simulink model "sampleModel1896"  (R2023a)
settings: Solver=VariableStepAuto  StartTime=0.0  StopTime=10.0  RelTol=1e-3
libraries: hdlsllib x5
settings Model: Creator=user1  LastModifiedBy=user1

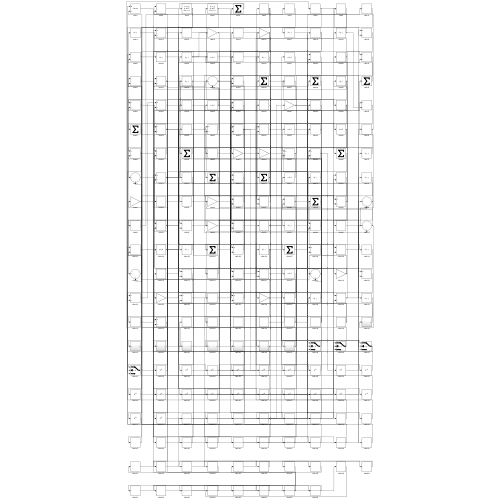
[thumbnail: Simulink's stored preview of the top-level diagram]
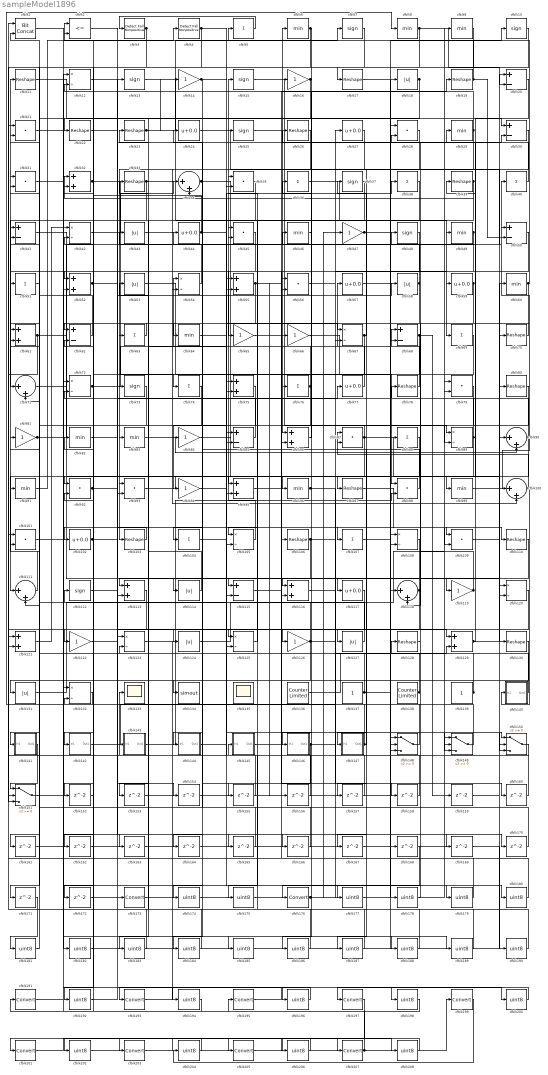
== system sampleModel1896 ==
  cfblk1 : hdlsllib/Logic and Bit Operations/Bit Concat  numInputs=2
  cfblk{7,10,13,15,25,37,48,73,112} (9 alike) : Signum
  cfblk{34,71,90,100,111,118} (6 alike) : Sum  Inputs=|++
  cfblk{21,28,31,35,45,56,79,87,92..93,98,101,109} (13 alike) : DotProduct  OutDataTypeStr=Inherit: Inherit via internal rule
  cfblk{24,27,44,57,59,77,102,117} (8 alike) : Bias  Bias=0.0  SaturateOnIntegerOverflow=off
  cfblk{11,17,19,22..23,26,33,39,70,78,80,97,103,106,110,128,130} (17 alike) : Reshape
  cfblk{5,36,38,40,51,63,69,74,76,88,104,107} (12 alike) : Sum  Inputs=+
  cfblk{12,42,54,67,72,89,105,108,120,123,125,132} (12 alike) : Product  Inputs=*/  RndMeth=Zero  SaturateOnIntegerOverflow=on
  cfblk{32,52,55,61,75,86,95,113,116,121,129} (11 alike) : Sum
  cfblk{18,43,53,58,114,124,127,131} (8 alike) : Abs  SaturateOnIntegerOverflow=off
  cfblk{20,30,41,50,62,68,85,115} (8 alike) : Sum  Inputs=+-
  cfblk{14,16,47,65..66,81,84,94,119,122,126} (11 alike) : Gain
  cfblk133 : Scope
  cfblk134 : ToWorkspace  VariableName=simout  SaveFormat=Timeseries  SampleTime=-1
  cfblk135 : Scope
      settings: Floating=on
  cfblk136 : hdlsllib/Sources/Counter Limited  uplimit=7  tsamp=-1
  cfblk137 : Constant  SampleTime=-1
  cfblk138 : hdlsllib/Sources/Counter Limited  uplimit=7  tsamp=-1
  cfblk139 : Constant  SampleTime=-1
  cfblk140 : Subsystem
      settings: LibrarySourceBlock=|
      | hdlsllib/Ports &
      | Subsystems/Subsystem
  cfblk141 : Subsystem
      settings: LibrarySourceBlock=|
      | hdlsllib/Ports &
      | Subsystems/Subsystem
  cfblk142 : Subsystem
      settings: LibrarySourceBlock=|
      | hdlsllib/Ports &
      | Subsystems/Subsystem
  cfblk143 : Subsystem
      settings: LibrarySourceBlock=|
      | hdlsllib/Ports &
      | Subsystems/Subsystem
  cfblk144 : Subsystem
      settings: LibrarySourceBlock=|
      | hdlsllib/Ports &
      | Subsystems/Subsystem
  cfblk145 : Subsystem
      settings: LibrarySourceBlock=|
      | hdlsllib/Ports &
      | Subsystems/Subsystem
  cfblk146 : Subsystem
      settings: LibrarySourceBlock=|
      | hdlsllib/Ports &
      | Subsystems/Subsystem
  cfblk147 : Subsystem
      settings: LibrarySourceBlock=|
      | hdlsllib/Ports &
      | Subsystems/Subsystem
  cfblk{148..151} (4 alike) : Switch  SaturateOnIntegerOverflow=off  InputSameDT=off
  cfblk{152..172} (21 alike) : Delay  SampleTime=1
  cfblk{173,176,191,193,195,197,199,201,203,205,207} (11 alike) : DataTypeConversion  SaturateOnIntegerOverflow=off  RndMeth=Floor
  cfblk{174..175,177..190,192,194,196,198,200,202,204,206,208} (25 alike) : DataTypeConversion  OutDataTypeStr=uint8  SaturateOnIntegerOverflow=off  RndMeth=Floor
  cfblk2 : RelationalOperator  Operator=<=  OutDataTypeStr=boolean  InputSameDT=off
  cfblk{6,8..9,29,46,49,60,64,82..83,91,96,99} (13 alike) : MinMax
  cfblk3 : hdlsllib/Logic and Bit Operations/Detect Fall Nonpositive  vinit=0  OutDataTypeStr=boolean
  cfblk4 : hdlsllib/Logic and Bit Operations/Detect Fall Nonpositive  vinit=0  OutDataTypeStr=boolean
  wires:
  cfblk68/1 -> cfblk105/2, cfblk159/1
  cfblk54/1 -> cfblk22/1
  cfblk32/1 -> cfblk74/1, cfblk162/1
  cfblk105/1 -> cfblk15/1
  cfblk98/1 -> cfblk44/1
  cfblk121/1 -> cfblk42/1
  cfblk128/1 -> cfblk57/1
  cfblk30/1 -> cfblk108/2
  cfblk91/1 -> cfblk4/1
  cfblk84/1 -> cfblk96/1
  cfblk53/1 -> cfblk98/1
  cfblk137/1 -> cfblk18/1, cfblk32/1
  cfblk26/1 -> cfblk103/1
  cfblk114/1 -> cfblk53/1
  cfblk61/1 -> cfblk115/1, cfblk121/2
  cfblk70/1 -> cfblk63/1
  cfblk93/1 -> cfblk95/1
  cfblk34/1 -> cfblk148/2, cfblk120/2
  cfblk25/1 -> cfblk86/1
  cfblk5/1 -> cfblk3/1
  cfblk138/1 -> cfblk48/1, cfblk134/1, cfblk81/1
  cfblk60/1 -> cfblk5/1, cfblk118/2
  cfblk99/1 -> cfblk40/1
  cfblk23/1 -> cfblk7/1, cfblk14/1, cfblk30/2
  cfblk41/1 -> cfblk97/1
  cfblk92/1 -> cfblk13/1, cfblk107/1
  cfblk81/1 -> cfblk20/1, cfblk61/2
  cfblk111/1 -> cfblk11/1
  cfblk20/1 -> cfblk99/1
  cfblk49/1 -> cfblk65/1, cfblk45/2
  cfblk71/1 -> cfblk119/1
  cfblk97/1 -> cfblk110/1
  cfblk9/1 -> cfblk126/1
  cfblk89/1 -> cfblk39/1, cfblk144/1(In1), cfblk36/1
  cfblk87/1 -> cfblk130/1, cfblk104/1, cfblk84/1
  cfblk17/1 -> cfblk89/1
  cfblk140/1(Out1) -> cfblk78/1
  cfblk15/1 -> cfblk89/2
  cfblk8/1 -> cfblk20/2, cfblk113/2
  cfblk145/1(Out1) -> cfblk106/1
  cfblk28/1 -> cfblk176/1
  cfblk55/1 -> cfblk73/1, cfblk19/1, cfblk114/1, cfblk156/1
  cfblk64/1 -> cfblk95/2
  cfblk96/1 -> cfblk50/1, cfblk150/2
  cfblk36/1 -> cfblk69/1
  cfblk90/1 -> cfblk43/1, cfblk157/1
  cfblk109/1 -> cfblk80/1
  cfblk150/1 -> cfblk133/1
  cfblk100/1 -> cfblk140/1(In1), cfblk87/2
  cfblk73/1 -> cfblk83/1
  cfblk76/1 -> cfblk23/1, cfblk116/2
  cfblk63/1 -> cfblk62/1
  cfblk13/1 -> cfblk88/1
  cfblk77/1 -> cfblk54/1
  cfblk40/1 -> cfblk6/1
  cfblk125/1 -> cfblk45/1
  cfblk35/1 -> cfblk71/1
  cfblk119/1 -> cfblk116/1, cfblk68/2
  cfblk118/1 -> cfblk117/1, cfblk151/3
  cfblk115/1 -> cfblk98/2
  cfblk124/1 -> cfblk9/1
  cfblk50/1 -> cfblk86/2
  cfblk122/1 -> cfblk46/1
  cfblk127/1 -> cfblk112/1
  cfblk38/1 -> cfblk125/1
  cfblk129/1 -> cfblk60/1, cfblk29/1
  cfblk106/1 -> cfblk113/1, cfblk149/3, cfblk153/1
  cfblk45/1 -> cfblk51/1
  cfblk131/1 -> cfblk75/1
  cfblk112/1 -> cfblk77/1
  cfblk48/1 -> cfblk125/2
  cfblk42/1 -> cfblk34/1
  cfblk88/1 -> cfblk111/1
  cfblk10/1 -> cfblk17/1
  cfblk142/1(Out1) -> cfblk27/1
  cfblk46/1 -> cfblk146/1(In1)
  cfblk108/1 -> cfblk127/1
  cfblk148/1 -> cfblk33/1
  cfblk58/1 -> cfblk92/1, cfblk24/1
  cfblk75/1 -> cfblk94/1
  cfblk146/1(Out1) -> cfblk129/2, cfblk164/1
  cfblk132/1 -> cfblk8/1
  cfblk102/1 -> cfblk129/1, cfblk124/1, cfblk170/1
  cfblk4/1 -> cfblk141/1(In1), cfblk67/1
  cfblk86/1 -> cfblk16/1
  cfblk33/1 -> cfblk85/2, cfblk172/1
  cfblk83/1 -> cfblk90/2
  cfblk51/1 -> cfblk91/1
  cfblk72/1 -> cfblk55/2, cfblk58/1, cfblk25/1
  cfblk47/1 -> cfblk49/1, cfblk169/1
  cfblk67/1 -> cfblk122/1, cfblk37/1
  cfblk29/1 -> cfblk12/2, cfblk167/1
  cfblk78/1 -> cfblk35/1
  cfblk44/1 -> cfblk2/1, cfblk150/3
  cfblk82/1 -> cfblk109/1
  cfblk59/1 -> cfblk105/1, cfblk187/1
  cfblk19/1 -> cfblk2/2, cfblk50/2
  cfblk27/1 -> cfblk54/2
  cfblk147/1(Out1) -> cfblk31/1, cfblk87/1
  cfblk104/1 -> cfblk75/2
  cfblk37/1 -> cfblk93/1
  cfblk65/1 -> cfblk26/1
  cfblk18/1 -> cfblk41/1, cfblk52/2
  cfblk7/1 -> cfblk142/1(In1)
  cfblk136/1 -> cfblk128/1
  cfblk130/1 -> cfblk131/1
  cfblk39/1 -> cfblk93/2, cfblk32/2
  cfblk62/1 -> cfblk41/2
  cfblk141/1(Out1) -> cfblk151/1
  cfblk85/1 -> cfblk72/2
  cfblk56/1 -> cfblk59/1
  cfblk24/1 -> cfblk120/1
  cfblk144/1(Out1) -> cfblk38/1
  cfblk126/1 -> cfblk71/2, cfblk150/1, cfblk171/1
  cfblk3/1 -> cfblk52/1, cfblk151/2
  cfblk52/1 -> cfblk143/1(In1), cfblk166/1
  cfblk143/1(Out1) -> cfblk66/1
  cfblk6/1 -> cfblk111/2, cfblk61/1, cfblk76/1
  cfblk103/1 -> cfblk102/1
  cfblk16/1 -> cfblk35/2, cfblk184/1
  cfblk110/1 -> cfblk147/1(In1)
  cfblk149/1 -> cfblk132/2
  cfblk139/1 -> cfblk68/1, cfblk92/2
  cfblk11/1 -> cfblk30/1
  cfblk107/1 -> cfblk10/1
  cfblk2/1 -> cfblk109/2
  cfblk66/1 -> cfblk118/1
  cfblk14/1 -> cfblk115/2, cfblk64/1
  cfblk43/1 -> cfblk100/2
  cfblk113/1 -> cfblk152/1
  cfblk152/1 -> cfblk62/2
  cfblk153/1 -> cfblk56/2
  cfblk22/1 -> cfblk154/1
  cfblk154/1 -> cfblk108/1
  cfblk80/1 -> cfblk155/1
  cfblk155/1 -> cfblk132/1
  cfblk156/1 -> cfblk85/1
  cfblk157/1 -> cfblk55/1
  cfblk116/1 -> cfblk158/1
  cfblk158/1 -> cfblk121/1
  cfblk159/1 -> cfblk90/1
  cfblk95/1 -> cfblk160/1
  cfblk160/1 -> cfblk72/1
  cfblk74/1 -> cfblk161/1
  cfblk161/1 -> cfblk148/1
  cfblk162/1 -> cfblk149/2
  cfblk151/1 -> cfblk163/1
  cfblk163/1 -> cfblk149/1
  cfblk164/1 -> cfblk100/1
  cfblk12/1 -> cfblk165/1
  cfblk165/1 -> cfblk42/2
  cfblk166/1 -> cfblk34/2
  cfblk170/1 -> cfblk31/2
  cfblk172/1 -> cfblk148/3
  cfblk117/1 -> cfblk174/1
  cfblk174/1 -> cfblk79/1
  cfblk120/1 -> cfblk175/1
  cfblk175/1 -> cfblk79/2
  cfblk176/1 -> cfblk67/2, cfblk47/1
  cfblk94/1 -> cfblk177/1
  cfblk177/1 -> cfblk28/1
  cfblk57/1 -> cfblk178/1
  cfblk178/1 -> cfblk28/2
  cfblk1/1 -> cfblk179/1
  cfblk179/1 -> cfblk56/1
  cfblk167/1 -> cfblk180/1
  cfblk180/1 -> cfblk1/1
  cfblk171/1 -> cfblk181/1
  cfblk181/1 -> cfblk1/2
  cfblk101/1 -> cfblk182/1
  cfblk182/1 -> cfblk168/1
  cfblk69/1 -> cfblk183/1
  cfblk183/1 -> cfblk101/1
  cfblk184/1 -> cfblk101/2
  cfblk21/1 -> cfblk185/1
  cfblk185/1 -> cfblk70/1
  cfblk168/1 -> cfblk186/1
  cfblk186/1 -> cfblk21/1
  cfblk187/1 -> cfblk21/2
  cfblk123/1 -> cfblk188/1
  cfblk188/1 -> cfblk145/1(In1)
  cfblk31/1 -> cfblk189/1
  cfblk189/1 -> cfblk123/1
  cfblk169/1 -> cfblk190/1
  cfblk190/1 -> cfblk123/2
  cfblk79/1 -> cfblk192/1
  cfblk192/1 -> cfblk173/1
  cfblk173/1 -> cfblk194/1
  cfblk194/1 -> cfblk191/1
  cfblk191/1 -> cfblk196/1
  cfblk196/1 -> cfblk193/1
  cfblk193/1 -> cfblk198/1
  cfblk198/1 -> cfblk195/1
  cfblk195/1 -> cfblk200/1
  cfblk200/1 -> cfblk197/1
  cfblk197/1 -> cfblk202/1
  cfblk202/1 -> cfblk199/1
  cfblk199/1 -> cfblk204/1
  cfblk204/1 -> cfblk201/1
  cfblk205/1 -> cfblk207/1
  cfblk201/1 -> cfblk206/1
  cfblk206/1 -> cfblk203/1
  cfblk207/1 -> cfblk82/1, cfblk12/1
  cfblk203/1 -> cfblk208/1
  cfblk208/1 -> cfblk205/1

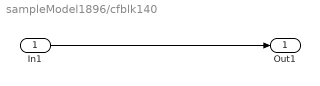
== system sampleModel1896/cfblk140 ==
  In1 : Inport
  Out1 : Outport
  wires:
  In1/1 -> Out1/1

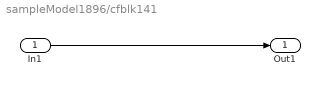
== system sampleModel1896/cfblk141 ==
  In1 : Inport
  Out1 : Outport
  wires:
  In1/1 -> Out1/1

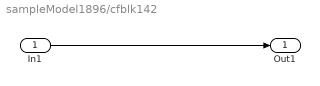
== system sampleModel1896/cfblk142 ==
  In1 : Inport
  Out1 : Outport
  wires:
  In1/1 -> Out1/1

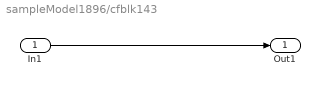
== system sampleModel1896/cfblk143 ==
  In1 : Inport
  Out1 : Outport
  wires:
  In1/1 -> Out1/1

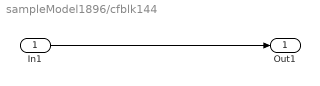
== system sampleModel1896/cfblk144 ==
  In1 : Inport
  Out1 : Outport
  wires:
  In1/1 -> Out1/1

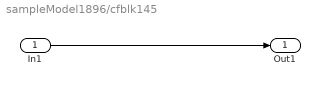
== system sampleModel1896/cfblk145 ==
  In1 : Inport
  Out1 : Outport
  wires:
  In1/1 -> Out1/1

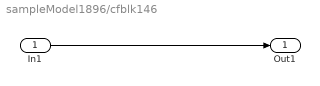
== system sampleModel1896/cfblk146 ==
  In1 : Inport
  Out1 : Outport
  wires:
  In1/1 -> Out1/1

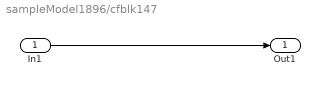
== system sampleModel1896/cfblk147 ==
  In1 : Inport
  Out1 : Outport
  wires:
  In1/1 -> Out1/1
